simulink model "assignment2a_GFM"  (R2024b)
settings: Solver=VariableStepAuto  StartTime=0.0  StopTime=0.15  RelTol=1e-3
libraries: spsIGBTDiodeLib x6, spsDCVoltageSourceLib x1, spsGroundLib x1, spsPower3phInstantaneousLib x1, spsThreePhaseParallelRLCBranchLib x1, spsThreePhaseSeriesRLCBranchLib x1, spsThreePhaseSeriesRLCLoadLib x1, spsThreePhaseVIMeasurementLib x1, spsTriangleGeneratorLib x1, spsVoltageMeasurementLib x1, spsdq0toabcLib x1, spspowerguiLib x1
settings Model: Creator=alexapf.stu  LastModifiedBy=alexapf.stu

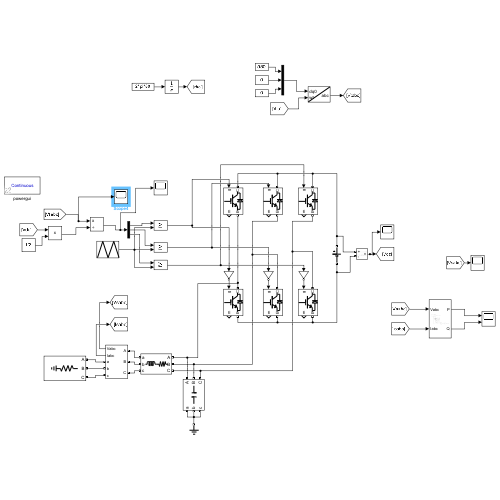
[thumbnail: Simulink's stored preview of the top-level diagram]
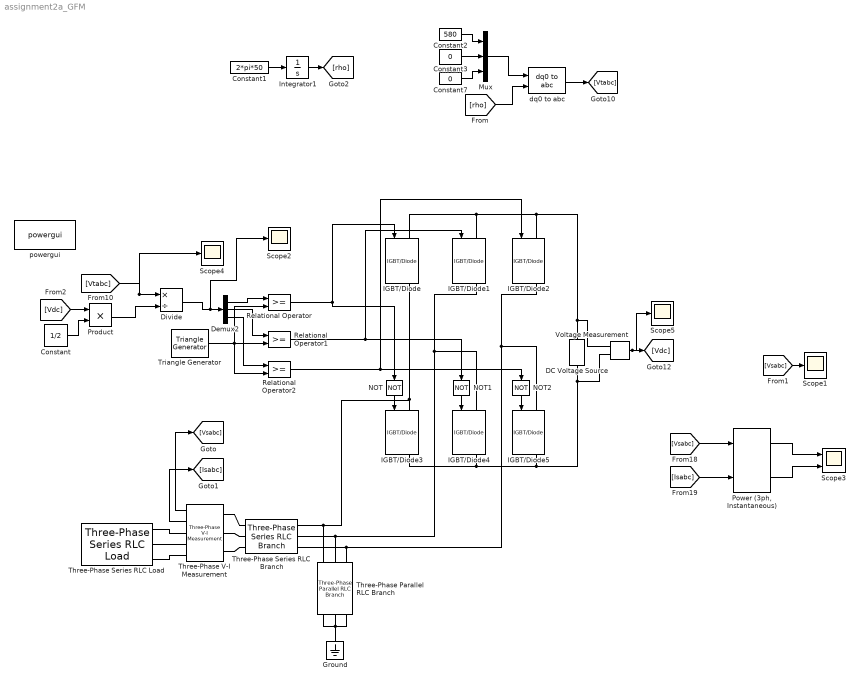
== system assignment2a_GFM ==
  Constant : Constant  Value=1/2
  Constant1 : Constant  Value=2*pi*50
  Constant2 : Constant  Value=580
  Constant3 : Constant  Value=0
  Constant7 : Constant  Value=0
  DC Voltage Source : spsDCVoltageSourceLib/DC Voltage Source  Amplitude=1000  Measurements=None
  Demux2 : Demux  Outputs=3
  Divide : Product  Inputs=*/
  Ground : spsGroundLib/Ground  LConnTagsString=a
  IGBT/Diode{,1..5} (6 alike) : spsIGBTDiodeLib/IGBT//Diode  Ron=1e-3  Rs=1e5  Cs=inf  Measurements=on
  Integrator1 : Integrator
  Mux : Mux  Inputs=3
  NOT : Logic  Operator=NOT  IconShape=distinctive  AllPortsSameDT=off  OutDataTypeStr=boolean
  NOT1 : Logic  Operator=NOT  IconShape=distinctive  AllPortsSameDT=off  OutDataTypeStr=boolean
  NOT2 : Logic  Operator=NOT  IconShape=distinctive  AllPortsSameDT=off  OutDataTypeStr=boolean
  "Power (3ph, Instantaneous)" : spsPower3phInstantaneousLib/Power (3ph, Instantaneous)
  Product : Product
  Relational Operator : RelationalOperator  OutDataTypeStr=boolean  RndMeth=Simplest  InputSameDT=off
  Relational Operator1 : RelationalOperator  OutDataTypeStr=boolean  RndMeth=Simplest  InputSameDT=off
  Relational Operator2 : RelationalOperator  OutDataTypeStr=boolean  RndMeth=Simplest  InputSameDT=off
  Scope{1..2,4..5} (4 alike) : Scope
  Scope3 : Scope  NumInputPorts=2
  Three-Phase Parallel RLC Branch : spsThreePhaseParallelRLCBranchLib/Three-Phase Parallel RLC Branch  LConnTagsString=A|B|C  RConnTagsString=A|B|C  BranchType=C  Resistance=1  Inductance=1e-3  Capacitance=189e-6  Measurements=None
  Three-Phase Series RLC Branch : spsThreePhaseSeriesRLCBranchLib/Three-Phase Series RLC Branch  LConnTagsString=A|B|C  RConnTagsString=A|B|C  BranchType=RL  Resistance=1.6e-3  Inductance=1.6e-3  Capacitance=1e-6  Measurements=Branch voltages and currents
  Three-Phase Series RLC Load : spsThreePhaseSeriesRLCLoadLib/Three-Phase Series RLC Load  LConnTagsString=A|B|C  Configuration=Y (grounded)  NominalVoltage=580  Vabc=[1e3 1e3 1e3]  Vabcp=[1e3 1e3 1e3]  NominalFrequency=50  UnbalancedPower=off  ActivePower=100e3  InductivePower=0  CapacitivePower=0  Pabc=[10e3 9e3 11e3]  QLabc=[100 90 110]  QCabc=[100 90 110]  Pabcp=[10e3 9e3 11e3]  QLabcp=[100 90 110]  QCabcp=[100 90 110]  Measurements=Branch voltages and currents  LoadType=constant Z
  Three-Phase V-I Measurement : spsThreePhaseVIMeasurementLib/Three-Phase V-I Measurement  VoltageMeasurement=phase-to-ground  SetLabelV=off  LabelV=Vabc  Vpu=off  VpuLL=off  CurrentMeasurement=yes  SetLabelI=off  LabelI=Iabc  Ipu=off  Pbase=100e3  Vbase=580  OutputType=Complex  PhasorSimulation=off  PSBequivalent=0
  Triangle Generator : spsTriangleGeneratorLib/Triangle Generator  Freq=3060  Phase=0  Ts=0
  Voltage Measurement : spsVoltageMeasurementLib/Voltage Measurement  PhasorSimulation=off  OutputType=Complex  PSBequivalent=0
  dq0 to abc : spsdq0toabcLib/dq0 to abc  Alignment=90 degrees behind phase A axis
  powergui : spspowerguiLib/powergui  Priority=1  SimulationMode=Continuous  SampleTime=50e-6  frequency=60  Iterations=50  frequencyindice=0  Pbase=100e6  ErrMax=1e-4  UnitsV=kV  UnitsW=MW  buscounter=0  FunctionMessages=off  echomessages=off  EnableUseOfTLC=off  CurrentSourceSwitches=off  DisableSnubberDevices=off  DisableRonSwitches=off  DisableVfSwitches=off  DisplayEquations=off  AutomaticDiscreteSolvers=off  SolverType=Tustin/Backward Euler (TBE)  Interpol=off  ExternalGateDelay=off  methode=off  Ts=100  x0status=blocks  SPID=on  SwTol=0  HookPort=off  NonlinearTolerance=1e-4  nMaxIteration=100  ContinueOnMaxIteration=off  RestoreLinks=warning  ResistiveCurrentMeasurement=off  Frange=[0:2:500]  Ylog=off  Xlog=on  ShowGrid=off  save=off  variable=ZData  structure=0  ZoomFFT=off  StartTime=0.0  cycles=1  DisplayStyle=1  fundamental=60  FreqAxis=off  MaxFrequency=1000  frequencyindicesteady=1  RmsSteady=1  display=off
  wires:
  [Vsabc] -> "Power (3ph, Instantaneous)"/1
  [Isabc] -> "Power (3ph, Instantaneous)"/2
  "Power (3ph, Instantaneous)"/1 -> Scope3/1
  "Power (3ph, Instantaneous)"/2 -> Scope3/2
  Three-Phase V-I Measurement/2 -> [Isabc]
  Demux2/2 -> Relational Operator1/1
  Demux2/3 -> Relational Operator2/1
  Demux2/1 -> Relational Operator/1
  Three-Phase V-I Measurement/1 -> [Vsabc]
  Triangle Generator/1 -> Relational Operator2/2, Relational Operator1/2, Relational Operator/2
  Voltage Measurement/1 -> Scope5/1, [Vdc]
  Relational Operator/1 -> NOT/1, IGBT/Diode/1
  Relational Operator1/1 -> IGBT/Diode1/1, NOT1/1
  Relational Operator2/1 -> NOT2/1, IGBT/Diode2/1
  NOT/1 -> IGBT/Diode3/1
  NOT1/1 -> IGBT/Diode4/1
  NOT2/1 -> IGBT/Diode5/1
  dq0 to abc/1 -> [Vtabc]
  Constant3/1 -> Mux/2
  Constant2/1 -> Mux/1
  Constant7/1 -> Mux/3
  Mux/1 -> dq0 to abc/1
  Constant1/1 -> Integrator1/1
  Integrator1/1 -> [rho]
  [rho] -> dq0 to abc/2
  [Vsabc] -> Scope1/1
  [Vdc] -> Product/1
  Constant/1 -> Product/2
  Product/1 -> Divide/2
  [Vtabc] -> Scope4/1, Divide/1
  Divide/1 -> Scope2/1, Demux2/1
  connections:
  IGBT/Diode3/RConn1 -- DC Voltage Source/LConn1 -- Voltage Measurement/LConn2 -- IGBT/Diode5/RConn1 -- IGBT/Diode4/RConn1
  Voltage Measurement/LConn1 -- DC Voltage Source/RConn1 -- IGBT/Diode1/LConn1 -- IGBT/Diode/LConn1 -- IGBT/Diode2/LConn1
  IGBT/Diode3/LConn1 -- IGBT/Diode/RConn1 -- Three-Phase Series RLC Branch/LConn1 -- Three-Phase Parallel RLC Branch/LConn1
  IGBT/Diode1/RConn1 -- Three-Phase Series RLC Branch/LConn2 -- Three-Phase Parallel RLC Branch/LConn2 -- IGBT/Diode4/LConn1
  IGBT/Diode2/RConn1 -- Three-Phase Series RLC Branch/LConn3 -- Three-Phase Parallel RLC Branch/LConn3 -- IGBT/Diode5/LConn1
  Three-Phase Parallel RLC Branch/RConn3 -- Ground/LConn1 -- Three-Phase Parallel RLC Branch/RConn1 -- Three-Phase Parallel RLC Branch/RConn2
  Three-Phase V-I Measurement/LConn1 -- Three-Phase Series RLC Branch/RConn1
  Three-Phase V-I Measurement/LConn2 -- Three-Phase Series RLC Branch/RConn2
  Three-Phase V-I Measurement/LConn3 -- Three-Phase Series RLC Branch/RConn3
  Three-Phase Series RLC Load/LConn2 -- Three-Phase V-I Measurement/RConn2
  Three-Phase Series RLC Load/LConn1 -- Three-Phase V-I Measurement/RConn1
  Three-Phase Series RLC Load/LConn3 -- Three-Phase V-I Measurement/RConn3
